simulink model "Lab2_lqc"  (R2023b)
settings: Solver=FixedStepAuto  StartTime=0.0  StopTime=30  FixedStep=.01  RelTol=1e-3
undefined symbols (not defined in the file or in its folder): A, B, C, mult_lqc
settings Model: Creator=Connor Emmons  LastModifiedBy=Connor Emmons

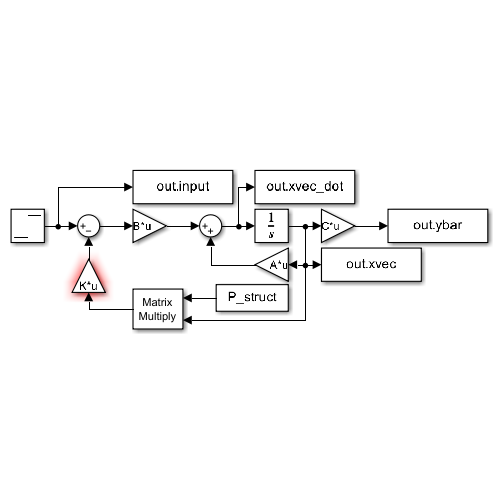
[thumbnail: Simulink's stored preview of the top-level diagram]
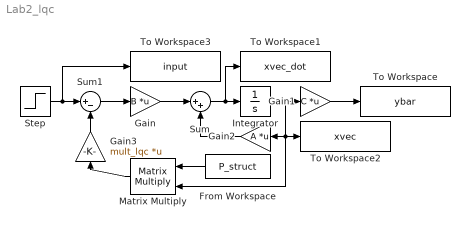
== system Lab2_lqc ==
  From Workspace : FromWorkspace  VariableName=P_struct
  Gain : Gain  Gain=B  Multiplication=Matrix(K*u)
  Gain1 : Gain  Gain=C  Multiplication=Matrix(K*u)
  Gain2 : Gain  Gain=A  Multiplication=Matrix(K*u)
  Gain3 : Gain  Gain=mult_lqc  Multiplication=Matrix(K*u)
  Integrator : Integrator
  Matrix Multiply : Product  Multiplication=Matrix(*)
  Step : Step  SampleTime=0
  Sum : Sum  Inputs=|++
  Sum1 : Sum  Inputs=|+-
  To Workspace : ToWorkspace  VariableName=ybar  SampleTime=-1
  To Workspace1 : ToWorkspace  VariableName=xvec_dot  SampleTime=-1
  To Workspace2 : ToWorkspace  VariableName=xvec  SampleTime=-1
  To Workspace3 : ToWorkspace  VariableName=input  SampleTime=-1
  wires:
  Gain/1 -> Sum/1
  Sum/1 -> To Workspace1/1, Integrator/1
  Integrator/1 -> Matrix Multiply/2, Gain2/1, To Workspace2/1, Gain1/1
  Gain2/1 -> Sum/2
  Gain1/1 -> To Workspace/1
  Step/1 -> To Workspace3/1, Sum1/1
  Sum1/1 -> Gain/1
  From Workspace/1 -> Matrix Multiply/1
  Gain3/1 -> Sum1/2
  Matrix Multiply/1 -> Gain3/1
